simulink model "self_balance_nonlinear"  (R2023b)
settings: Solver=ode4  StartTime=0.0  StopTime=5  FixedStep=0.0001  RelTol=1e-3
undefined symbols (not defined in the file): dt, I_body, I_wheel, initial_angle, M_body, M_wheel, r
libraries: slpidlib x1
settings Model: Creator=emamaker  LastModifiedBy=emamaker

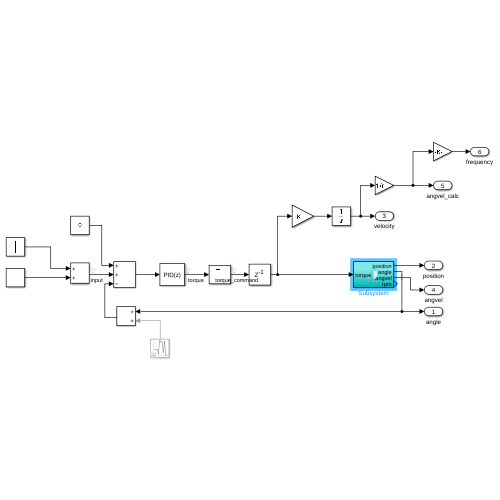
[thumbnail: Simulink's stored preview of the top-level diagram]
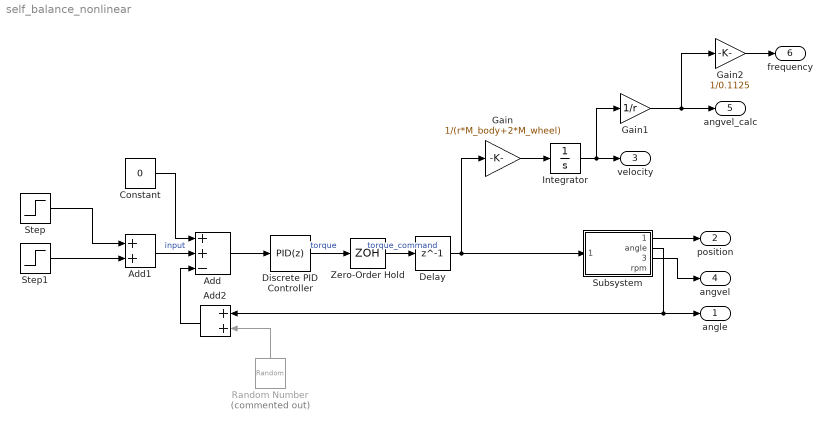
== system self_balance_nonlinear ==
  Add : Sum  Inputs=++-
  Add1 : Sum
  Add2 : Sum
  Constant : Constant  Value=0
  Delay : Delay  DelayLength=1
  Discrete PID Controller : slpidlib/PID Controller  Controller=PID  Form=Parallel  TimeDomain=Discrete-time  UseExternalTs=off  SampleTime=dt  IntegratorMethod=Forward Euler  FilterMethod=Forward Euler  ControllerParametersSource=internal  P=-3.5  I=-2  UseKiTs=off  D=-0.03  N=100  UseFilter=off  TunerSelectOption=Transfer Function Based (PID Tuner App)  InitialConditionSource=internal  InitialConditionForIntegrator=0  InitialConditionForFilter=0  DifferentiatorICPrevScaledInput=0  ExternalReset=none  TrackingMode=off  Kt=1  LimitOutput=off  SatLimitsSource=internal  UpperSaturationLimit=inf  LowerSaturationLimit=-inf  LinearizeAsGain=off  AntiWindupMode=none  Kb=1  LimitIntegrator=off  UpperIntegratorSaturationLimit=inf  LowerIntegratorSaturationLimit=-inf  POutMin=[]  POutMax=[]  IOutMin=[]  IOutMax=[]  DOutMin=[]  DOutMax=[]  NOutMin=[]  NOutMax=[]  SumOutMin=[]  SumOutMax=[]  SaturationOutMin=[]  SaturationOutMax=[]  PParamMin=[]  PParamMax=[]  IParamMin=[]  IParamMax=[]  DParamMin=[]  DParamMax=[]  NParamMin=[]  NParamMax=[]  KbParamMin=[]  KbParamMax=[]  KtParamMin=[]  KtParamMax=[]  KbOutMin=[]  KbOutMax=[]  KtOutMin=[]  KtOutMax=[]  IntegratorOutMin=[]  IntegratorOutMax=[]  FilterOutMin=[]  FilterOutMax=[]  SumI1OutMin=[]  SumI1OutMax=[]  SumI2OutMin=[]  SumI2OutMax=[]  SumI3OutMin=[]  SumI3OutMax=[]  SumI4OutMin=[]  SumI4OutMax=[]  SumDOutMin=[]  SumDOutMax=[]  DifferentiatorOutMin=[]  DifferentiatorOutMax=[]  FilterDiffOutCoefMin=[]  FilterDiffOutCoefMax=[]  ReciprocalOutMin=[]  ReciprocalOutMax=[]  SumDenOutMin=[]  SumDenOutMax=[]  SumNumOutMin=[]  SumNumOutMax=[]  DivideOutMin=[]  DivideOutMax=[]  UdiffTsProdOutMin=[]  UdiffTsProdOutMax=[]  NTsProdOutMin=[]  NTsProdOutMax=[]  UintegralTsProdOutMin=[]  UintegralTsProdOutMax=[]  UngainTsProdOutMin=[]  UngainTsProdOutMax=[]  ClampingZeroOutDataTypeStr=Inherit: Inherit via back propagation  ClampingZeroOutMin=[]  ClampingZeroOutMax=[]  FilterDenConstantOutDataTypeStr=Inherit: Inherit via back propagation  FilterDenConstantOutMin=[]  FilterDenConstantOutMax=[]  PCopyOutDataTypeStr=Inherit: Inherit via back propagation  PCopyOutMin=[]  PCopyOutMax=[]  NCopyOutDataTypeStr=Inherit: Inherit via back propagation  NCopyOutMin=[]  NCopyOutMax=[]  IntegratorContinuousStateAttributes=''  IntegratorStateMustResolveToSignalObject=off  IntegratorRTWStateStorageClass=Auto  FilterContinuousStateAttributes=''  FilterStateMustResolveToSignalObject=off  FilterRTWStateStorageClass=Auto  ParallelPVariant=InternalParameters  IdealPVariant=Disabled  IVariant=InternalParameters  DVariant=InternalParameters  IntegratorVariant=Discrete  SatVariant=Disabled  AWVariant=Passthrough  PCopyVariant=Disabled  TRVariant=Disabled  FdbkBlocksVariant=Forward  IdealPFdbkVariant=Disabled  SatFdbkVariant=Disabled  DerivativeFilterVariant=Differentiator  NVariant=Passthrough  NCopyVariant=Disabled_SignalSpec  FilterICVariant=InternalICsDifferentiator  IntegratorICVariant=InternalICs  ExternalResetVariant=Disabled  TRSumVariant=Passthrough  SumFdbkVariant=Disabled  SumVariant=Sum_PID  TsampFilterVariant=InternalTs  TsampNgainVariant=Passthrough  TsampIntegralVariant=Disabled_SignalSpec  ExternalSaturationOutDataTypeStr=Inherit: Same as second input
      settings: LibrarySourceBlock=simulink/Discrete/Discrete PID Controller
  Gain : Gain  Gain=1/(r*M_body+2*M_wheel)
  Gain1 : Gain  Gain=1/r
  Gain2 : Gain  Gain=1/0.1125
  Integrator : Integrator
  Random Number : RandomNumber  Commented=on  Variance=0.0001  SampleTime=dt*10
  Step : Step  After=initial_angle  SampleTime=dt
  Step1 : Step  Time=1.01  After=-initial_angle  SampleTime=dt
  Subsystem : Subsystem
  Zero-Order Hold : ZeroOrderHold  SampleTime=-1
  angle : Outport
  position : Outport  Port=2
  velocity : Outport  Port=3
  angvel : Outport  Port=4
  angvel_calc : Outport  Port=5
  frequency : Outport  Port=6
  wires:
  Subsystem/2(angle) -> Add2/1, angle/1
  Add1/1 -> Add/2  "input"
  Step/1 -> Add1/1
  Constant/1 -> Add/1
  Add/1 -> Discrete PID Controller/1
  Subsystem/1(position) -> position/1
  Step1/1 -> Add1/2
  Discrete PID Controller/1 -> Zero-Order Hold/1  "torque"
  Add2/1 -> Add/3
  Random Number/1 -> Add2/2
  Zero-Order Hold/1 -> Delay/1  "torque_command"
  Gain/1 -> Integrator/1
  Integrator/1 -> Gain1/1, velocity/1
  Delay/1 -> Gain/1, Subsystem/1(torque)
  Subsystem/3(angvel) -> angvel/1
  Gain1/1 -> Gain2/1, angvel_calc/1
  Gain2/1 -> frequency/1

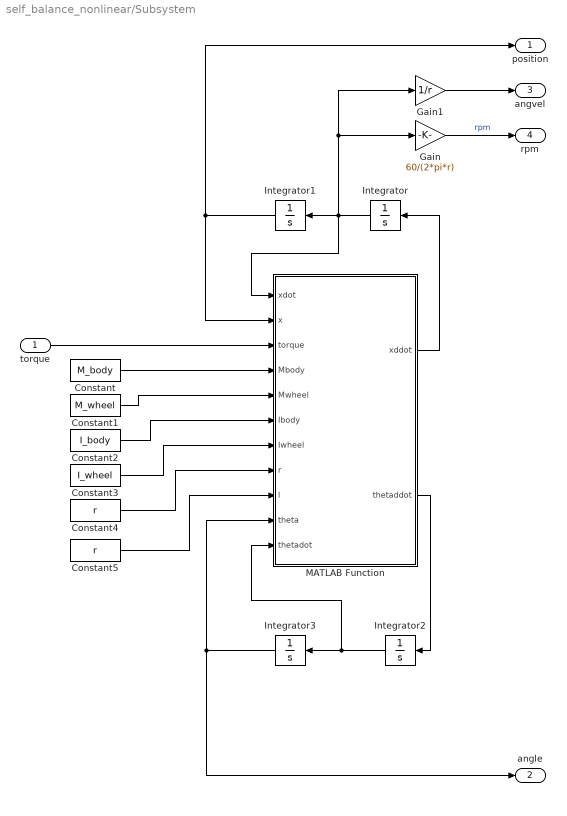
== system self_balance_nonlinear/Subsystem ==
  torque : Inport
  Constant : Constant  Value=M_body
  Constant1 : Constant  Value=M_wheel
  Constant2 : Constant  Value=I_body
  Constant3 : Constant  Value=I_wheel
  Constant4 : Constant  Value=r
  Constant5 : Constant  Value=r
  Gain : Gain  Gain=60/(2*pi*r)
  Gain1 : Gain  Gain=1/r
  Integrator{,1..3} (4 alike) : Integrator
  MATLAB Function : MATLAB Function  TreatAsAtomicUnit=on
  position : Outport
  angle : Outport  Port=2
  angvel : Outport  Port=3
  rpm : Outport  Port=4
  wires:
  MATLAB Function/1(xddot) -> Integrator/1
  Integrator1/1 -> position/1, MATLAB Function/2(x)
  Integrator2/1 -> Integrator3/1, MATLAB Function/11(thetadot)
  MATLAB Function/2(thetaddot) -> Integrator2/1
  torque/1 -> MATLAB Function/3(torque)
  Integrator3/1 -> MATLAB Function/10(theta), angle/1
  Integrator/1 -> Integrator1/1, Gain1/1, Gain/1, MATLAB Function/1(xdot)
  Constant/1 -> MATLAB Function/4(Mbody)
  Constant1/1 -> MATLAB Function/5(Mwheel)
  Constant2/1 -> MATLAB Function/6(Ibody)
  Constant3/1 -> MATLAB Function/7(Iwheel)
  Constant4/1 -> MATLAB Function/8(r)
  Constant5/1 -> MATLAB Function/9(l)
  Gain/1 -> rpm/1  "rpm"
  Gain1/1 -> angvel/1

== matlab function self_balance_nonlinear/Subsystem/MATLAB Function ==
  data: xdot input; xddot output; x input; torque input; Mbody input; Mwheel input; Ibody input; Iwheel input; r input; l input; thetaddot output; theta input; thetadot input
function [xddot, thetaddot]= fcn(xdot, x, torque, Mbody, Mwheel, Ibody, Iwheel, r, l,theta, thetadot)

% friction
b = 0.1;
% acceleration of gravity
g = 9.81;

%{
% commonly seen coeff
coeff_Ib_mbl2 = I_body + M_body*(l^2)
coeff_mb_Iw_mw = M_body + 2*I_wheel/(r^2) + 2*M_wheel
coeff_mb_l = M_body*l
coeff_mb2_l2 = coeff_mb_l^2

xddot = (1/coeff_mb_Iw_mw) * ( -coeff_mb_l*thetaddot_old*cos(theta)) + coeff_mb_l*(thetadot^2)*sin(theta) + torque/r - xdot*b*(r^2);
thetaddot = 1/(coeff_Ib_mbl2) * (-coeff_mb_l*xddot_old*cos(theta) + coeff_mb_l*g*sin(theta) - torque);
%}

sigma1 = Mbody*l*cos(theta);
sigma2 = Mbody+2*Mwheel+2*Iwheel/(r^2);
sigma3 = Mbody*l*(thetadot^2)*sin(theta);

xddot_den_num = (Mbody * l^2 + Ibody)*(Mbody + 2*Mwheel + 2*Iwheel/(r^2));
xddot_den = sigma1 - xddot_den_num / sigma1;
xddot_num = torque - Mbody*g*l*sin(theta) + ((Mbody*(l^2)+Ibody)*(torque/r - b*(r^2)*xdot + Mbody*l*(thetadot^2)*sin(theta)))/ sigma1;
xddot = -xddot_num / xddot_den;


thetaddot_num = torque/r - b*(r^2)*xdot + (torque - Mbody*g*l*sin(theta) + ( (Mbody*(l^2) + Ibody)*(torque/r - b*(r^2)*xdot + sigma3) )/sigma1 ) / (sigma1 - (Mbody*(l^2)+Ibody*sigma2)/sigma1 );
thetaddot = thetaddot_num / sigma1;
